simulink model "p1_MCU"  (R2023a)
settings: Solver=FixedStepDiscrete  StartTime=0.0  StopTime=inf  FixedStep=Ts_MCU  RelTol=1e-3  EnableMultiTasking=on
PreLoadFcn:
  | p1_params_new
  | spiDataDefinition
InitFcn:
  | mbd_s32k_consistency_checks(bdroot(gcs));
undefined symbols (not defined in the file or in its folder): ack, cpr_handwheel, cpr_steering, Discrete, DriverInput, DrivetrainLeft, DrivetrainRight, LQFP, MPU_IO, n_handwheel, n_steering, p1data, p1params, param, sr, steering_limit, SteeringLeft, SteeringRight, Time, Ts_MCU, wc, WheelForceLeft, WheelForceRight
libraries: simulink x74, mbd_s32k1xx_ec_toolbox x58, Library_Drivetrain x5, Library_Steering x5, etargetslib x3, ctrlSharedLib x1
(part 1 of 4)
PreSaveFcn:
  | p1_params_new
  | spiDataDefinition
Description:
  | Sample code for extracting X,Y,Z components of acceleration from the on-board sensor.
  | 
  | Extra Modules (In addition to template defaults):
  | LPSPI0 (Accelerometer connection)
  | 
  | For more information, see our Accelerometer Guide:
  | https://www.audesseinc.com/labs/resources/accelerometer-guide/
  | 
  | Revision: 1.2
settings Model: LastModifiedBy=cbeal
settings SolverCC: AlgebraicLoopSolver=TrustRegion
settings DataIOCC: ExternalInput=off  InitialState=off  SaveOutput=off  SignalLogging=off  SaveTime=off
settings OptimizationCC: BlockReduction=off  DefaultParameterBehavior=Inlined  DefaultUnderspecifiedDataType=single  OptimizeBlockIOStorage=off  BufferReuse=off  GlobalBufferReuse=off  ExpressionFolding=off  EnableMemcpy=off  PassReuseOutputArgsAs=Individual arguments  LocalBlockOutputs=off  OptimizeDataStoreBuffers=off  BusAssignmentInplaceUpdate=off  OptimizationLevel=level0  EfficientTunableParamExpr=on
settings DebuggingCC: InheritedTsInSrcMsg=none  SingleTaskRateTransMsg=error  ParameterTunabilityLossMsg=error  UnconnectedInputMsg=error  UnconnectedOutputMsg=error  UnconnectedLineMsg=error  UnknownTsInhSupMsg=error  ArithmeticOperatorsInVariantConditions=warning
settings HardwareCC: ProdBitPerPointer=32  ProdBitPerSizeT=32  ProdBitPerPtrDiffT=32  ProdLargestAtomicInteger=Long  ProdLargestAtomicFloat=Double  ProdWordSize=32  ProdHWDeviceType=ARM Compatible->ARM Cortex
settings ModelReferenceCC: EnableRefExpFcnMdlSchedulingChecks=on
settings SFSimCC: MATLABDynamicMemAlloc=off  CustomCodeUndefinedFunction=UseInterfaceOnly
settings RTWCC: Description=Model Based Design Toolbox S32K1xx Code Generation Target  SystemTargetFile=mbd_s32k.tlc  MakeCommand=mbd_s32k_make_rtw COPY_MDLREF_INCLUDES=0  TemplateMakefile=mbd_s32k.tmf  GenerateReport=on  IncludeHyperlinkInReport=on  LaunchReport=on  GenerateTraceInfo=on  GenerateTraceReport=on  GenerateTraceReportSl=on  GenerateTraceReportSf=on  GenerateTraceReportEml=on  DLArmComputeVersion=19.05
settings CodeAppCC: ForceParamTrailComments=on  IgnoreCustomStorageClasses=off  OperatorAnnotations=on  SimulinkDataObjDesc=on  SFDataObjDesc=on  InsertBlockDesc=on  StateflowObjectComments=on
settings STFCustomTargetCC: MultiwordLength=256  ConcurrentExecutionCompliant=off  CombineOutputUpdateFcns=on  ERTCustomFileBanners=on  SupportContinuousTime=off  RemoveResetFunc=on  MATLABClassNameForMDSCustomization=Simulink.SoftwareTarget.ERTCustomization  GRTInterface=off  UseToolchainInfoCompliant=off  SystemTargetFile=mbd_s32k.tlc
settings ERTTargetCC: TargetLangStandard=C99 (ISO)  ParMdlRefBuildCompliant=off  CompOptLevelCompliant=off  ConcurrentExecutionCompliant=off  SupportNonInlinedSFcns=on  ModelStepFunctionPrototypeControlCompliant=off  CPPClassGenCompliant=off  UseToolchainInfoCompliant=off  InlinedParameterPlacement=NonHierarchical  ERTSrcFileBannerTemplate=mbd_ert_code_template.cgt  ERTHdrFileBannerTemplate=mbd_ert_code_template.cgt  ERTDataSrcFileTemplate=mbd_ert_code_template.cgt  ERTDataHdrFileTemplate=mbd_ert_code_template.cgt  ERTCustomFileTemplate=example_file_process.tlc

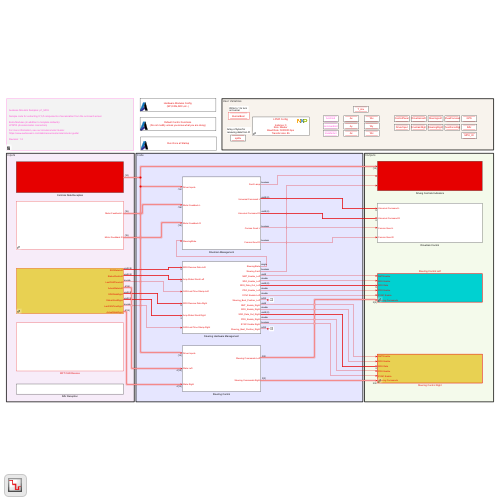
[thumbnail: Simulink's stored preview of the top-level diagram]
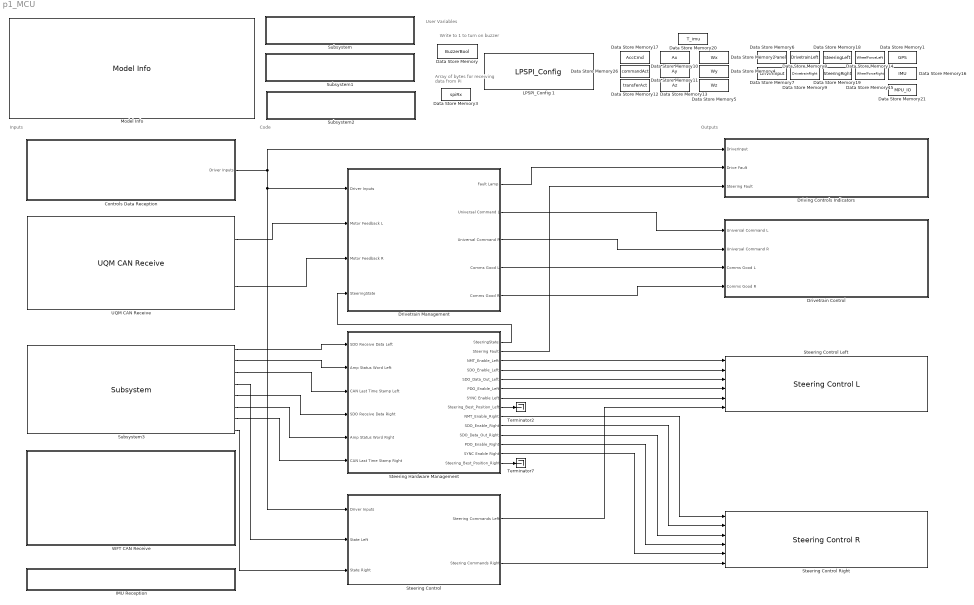
== system p1_MCU ==
  note: User Variables
  note: Write to 1 to turn on buzzer
  note: Inputs
  note: Code
  note: Outputs
  note: Array of bytes for receiving data from Pi
  " Controls Data Reception" : Subsystem  Priority=8
  Data Store Memory : DataStoreMemory  DataStoreName=BuzzerBool  ReadBeforeWriteMsg=warning  WriteAfterWriteMsg=warning  WriteAfterReadMsg=warning  ShowAdditionalParam=off  OutDataTypeStr=boolean
  Data Store Memory1 : DataStoreMemory  DataStoreName=GPS  ReadBeforeWriteMsg=warning  WriteAfterWriteMsg=warning  WriteAfterReadMsg=warning  InitialValue=zeros(p1data.gpsBytes,1)  ShowAdditionalParam=off  OutDataTypeStr=uint8
  Data Store Memory10 : DataStoreMemory  DataStoreName=Ax  ReadBeforeWriteMsg=warning  WriteAfterWriteMsg=warning  WriteAfterReadMsg=warning  InitialValue=[0]  ShowAdditionalParam=off  OutDataTypeStr=single
  Data Store Memory11 : DataStoreMemory  DataStoreName=Ay  ReadBeforeWriteMsg=warning  WriteAfterWriteMsg=warning  WriteAfterReadMsg=warning  InitialValue=[0]  ShowAdditionalParam=off  OutDataTypeStr=single
  Data Store Memory12 : DataStoreMemory  DataStoreName=transferAct  ReadBeforeWriteMsg=warning  WriteAfterWriteMsg=warning  WriteAfterReadMsg=warning  InitialValue=[1]  ShowAdditionalParam=off  OutDataTypeStr=boolean
  Data Store Memory13 : DataStoreMemory  DataStoreName=Az  ReadBeforeWriteMsg=warning  WriteAfterWriteMsg=warning  WriteAfterReadMsg=warning  InitialValue=[0]  ShowAdditionalParam=off  OutDataTypeStr=single
  Data Store Memory14 : DataStoreMemory  DataStoreName=WheelForceLeft  ReadBeforeWriteMsg=warning  WriteAfterWriteMsg=warning  WriteAfterReadMsg=warning  InitialValue=zeros(p1data.wftBytes,1)  ShowAdditionalParam=off  OutDataTypeStr=uint8
  Data Store Memory15 : DataStoreMemory  DataStoreName=WheelForceRight  ReadBeforeWriteMsg=warning  WriteAfterWriteMsg=warning  WriteAfterReadMsg=warning  InitialValue=zeros(p1data.wftBytes,1)  ShowAdditionalParam=off  OutDataTypeStr=uint8
  Data Store Memory16 : DataStoreMemory  DataStoreName=IMU  ReadBeforeWriteMsg=warning  WriteAfterWriteMsg=warning  WriteAfterReadMsg=warning  InitialValue=zeros(p1data.imuBytes,1)  ShowAdditionalParam=off  OutDataTypeStr=uint8
  Data Store Memory17 : DataStoreMemory  DataStoreName=AccCmd  ReadBeforeWriteMsg=warning  WriteAfterWriteMsg=warning  WriteAfterReadMsg=warning  InitialValue=[4436]  ShowAdditionalParam=off  OutDataTypeStr=uint16
  Data Store Memory18 : DataStoreMemory  DataStoreName=SteeringLeft  ReadBeforeWriteMsg=warning  WriteAfterWriteMsg=warning  WriteAfterReadMsg=warning  InitialValue=zeros(p1data.steeringBytes,1)  ShowAdditionalParam=off  OutDataTypeStr=uint8
  Data Store Memory19 : DataStoreMemory  DataStoreName=SteeringRight  ReadBeforeWriteMsg=warning  WriteAfterWriteMsg=warning  WriteAfterReadMsg=warning  InitialValue=zeros(p1data.steeringBytes,1)  ShowAdditionalParam=off  OutDataTypeStr=uint8
  Data Store Memory2 : DataStoreMemory  DataStoreName=Wx  ReadBeforeWriteMsg=warning  WriteAfterWriteMsg=warning  WriteAfterReadMsg=warning  InitialValue=[0]  ShowAdditionalParam=off  OutDataTypeStr=single
  Data Store Memory20 : DataStoreMemory  DataStoreName=T_imu  ReadBeforeWriteMsg=warning  WriteAfterWriteMsg=warning  WriteAfterReadMsg=warning  InitialValue=[0]  ShowAdditionalParam=off  OutDataTypeStr=single
  Data Store Memory21 : DataStoreMemory  DataStoreName=MPU_IO  ReadBeforeWriteMsg=warning  WriteAfterWriteMsg=warning  WriteAfterReadMsg=warning  InitialValue=zeros(p1data.mpuBytes,1)  ShowAdditionalParam=off  OutDataTypeStr=uint8
  Data Store Memory26 : DataStoreMemory  DataStoreName=commandAct  ReadBeforeWriteMsg=warning  WriteAfterWriteMsg=warning  WriteAfterReadMsg=warning  InitialValue=[0]  ShowAdditionalParam=off  OutDataTypeStr=boolean
  Data Store Memory3 : DataStoreMemory  DataStoreName=spiRx  ReadBeforeWriteMsg=warning  WriteAfterWriteMsg=warning  WriteAfterReadMsg=warning  InitialValue=zeros(p1data.spiBytes,1)  ShowAdditionalParam=off  OutDataTypeStr=uint8
  Data Store Memory4 : DataStoreMemory  DataStoreName=Wy  ReadBeforeWriteMsg=warning  WriteAfterWriteMsg=warning  WriteAfterReadMsg=warning  InitialValue=[0]  ShowAdditionalParam=off  OutDataTypeStr=single
  Data Store Memory5 : DataStoreMemory  DataStoreName=Wz  ReadBeforeWriteMsg=warning  WriteAfterWriteMsg=warning  WriteAfterReadMsg=warning  InitialValue=[0]  ShowAdditionalParam=off  OutDataTypeStr=single
  Data Store Memory6 : DataStoreMemory  DataStoreName=ControlPanel  ReadBeforeWriteMsg=warning  WriteAfterWriteMsg=warning  WriteAfterReadMsg=warning  InitialValue=zeros(p1data.controlPanelBytes,1)  ShowAdditionalParam=off  OutDataTypeStr=uint8
  Data Store Memory7 : DataStoreMemory  DataStoreName=DriverInput  ReadBeforeWriteMsg=warning  WriteAfterWriteMsg=warning  WriteAfterReadMsg=warning  InitialValue=zeros(p1data.driverInputBytes,1)  ShowAdditionalParam=off  OutDataTypeStr=uint8
  Data Store Memory8 : DataStoreMemory  DataStoreName=DrivetrainLeft  ReadBeforeWriteMsg=warning  WriteAfterWriteMsg=warning  WriteAfterReadMsg=warning  InitialValue=zeros(p1data.drivetrainBytes,1)  ShowAdditionalParam=off  OutDataTypeStr=uint8
  Data Store Memory9 : DataStoreMemory  DataStoreName=DrivetrainRight  ReadBeforeWriteMsg=warning  WriteAfterWriteMsg=warning  WriteAfterReadMsg=warning  InitialValue=zeros(p1data.drivetrainBytes,1)  ShowAdditionalParam=off  OutDataTypeStr=uint8
  Drivetrain Control : Subsystem
  Drivetrain Management : Subsystem
  Driving Controls Indicators : Subsystem
  IMU Reception : Subsystem
  LPSPI_Config 1 : mbd_s32k1xx_ec_toolbox/Communication Blocks/SPI Blocks/LPSPI_Config   Priority=0  InstanceNumber=0  Role=Master  BaudRate=5000000  ShowAdvanced=on  sin=PTE1: [LPSPI0_SIN | LPSPI Serial Data Input]  sout=PTE2: [LPSPI0_SOUT | LPSPI Serial Data Output]  sck=PTE0: [LPSPI0_SCK | LPSPI Serial Clock I/O]  pcs0=None  pcs1=None  pcs2=PTE6: [LPSPI0_PCS2 | Peripheral Chip Select 2]  pcs3=None  CPHA=1  CPOL=1  BitOrder=MSB first  TransferSize=8  WhichPCS=0  PCSPol=ActiveLow  ContinuousTransfer=off
  Model Info : simulink/Model-Wide Utilities/Model Info  Frame=on  DisplayStringWithTags=|  HorizontalTextAlignment=Left  LeftAlignmentValue=0.02
      | Audesse Simulink Samples: %<ModelName>
      | 
      | %<Description>
  Steering Control : Subsystem
  Steering Control Left : Library_Steering/Steering Control L  SystemSampleTime=-1  VariantActivationTime=update diagram  Latency=0  AutoFrameSizeCalculation=off
  Steering Control Right : Library_Steering/Steering Control R  SystemSampleTime=-1  VariantActivationTime=update diagram  Latency=0  AutoFrameSizeCalculation=off
  Steering Hardware Management : Subsystem
  Subsystem : Subsystem  Priority=1
      mask Display:
      | scl=1/4;
      | patch(scl*[0,52,90,54],scl*[16,55,146,146],[16/255,118/255,188/255],'bottom-left');
      | patch(scl*[0,27,82,77,68],scl*[16,0,42,62,69],[46/255,49/255,146/255],'bottom-left');
      | patch(scl*[89,125,90,68],scl*[16,16,146,91],[0,0,0],'bottom-left');
      | disp('Hardware Modules Config\n(SPI,CAN,ADC,etc..)');
  Subsystem1 : Subsystem
      mask Display:
      | scl=1/4;
      | patch(scl*[0,52,90,54],scl*[16,55,146,146],[16/255,118/255,188/255],'bottom-left');
      | patch(scl*[0,27,82,77,68],scl*[16,0,42,62,69],[46/255,49/255,146/255],'bottom-left');
      | patch(scl*[89,125,90,68],scl*[16,16,146,91],[0,0,0],'bottom-left');
      | disp('Default Control Functions\n(Do not modify unless you know what you are doing)');
  Subsystem2 : Subsystem  Priority=5
      mask Display:
      | scl=1/4;
      | patch(scl*[0,52,90,54],scl*[16,55,146,146],[16/255,118/255,188/255],'bottom-left');
      | patch(scl*[0,27,82,77,68],scl*[16,0,42,62,69],[46/255,49/255,146/255],'bottom-left');
      | patch(scl*[89,125,90,68],scl*[16,16,146,91],[0,0,0],'bottom-left');
      | disp('Run Once at Startup');
  Subsystem3 : Library_Steering/Subsystem  SystemSampleTime=-1  VariantActivationTime=update diagram  Latency=0  AutoFrameSizeCalculation=off
  Terminator2 : Terminator
  Terminator7 : Terminator
  UQM CAN Receive : Library_Drivetrain/UQM CAN Receive  SystemSampleTime=-1  VariantActivationTime=update diagram  Latency=0  AutoFrameSizeCalculation=off
  WFT CAN Receive : Subsystem
  wires:
  Drivetrain Management/5(Comms Good R) -> Drivetrain Control/4(Comms Good R)
  Drivetrain Management/4(Comms Good L) -> Drivetrain Control/3(Comms Good L)
  " Controls Data Reception"/1(Driver Inputs) -> Driving Controls Indicators/1(DriverInput), Steering Control/1(Driver Inputs), Drivetrain Management/1(Driver Inputs)
  Drivetrain Management/2(Universal Command L) -> Drivetrain Control/1(Universal Command L)
  UQM CAN Receive/2 -> Drivetrain Management/3(Motor Feedback R)
  Drivetrain Management/1(Fault Lamp) -> Driving Controls Indicators/2(Drive Fault)
  Drivetrain Management/3(Universal Command R) -> Drivetrain Control/2(Universal Command R)
  UQM CAN Receive/1 -> Drivetrain Management/2(Motor Feedback L)
  Subsystem3/1 -> Steering Hardware Management/1(SDO Receive Data Left)
  Subsystem3/2 -> Steering Hardware Management/2(Amp Status Word Left)
  Subsystem3/3 -> Steering Hardware Management/3(CAN Last Time Stamp Left)
  Subsystem3/4 -> Steering Control/2(State Left)
  Steering Hardware Management/2(Steering Fault) -> Driving Controls Indicators/3(Steering Fault)
  Steering Hardware Management/3(NMT_Enable_Left) -> Steering Control Left/1
  Steering Hardware Management/4(SDO_Enable_Left) -> Steering Control Left/2
  Steering Hardware Management/5(SDO_Data_Out_Left) -> Steering Control Left/3
  Steering Hardware Management/6(PDO_Enable_Left) -> Steering Control Left/4
  Steering Control/1(Steering Commands Left) -> Steering Control Left/6
  Steering Hardware Management/8(Steering_Best_Position_Left) -> Terminator2/1
  Subsystem3/6 -> Steering Hardware Management/5(Amp Status Word Right)
  Subsystem3/8 -> Steering Control/3(State Right)
  Subsystem3/5 -> Steering Hardware Management/4(SDO Receive Data Right)
  Subsystem3/7 -> Steering Hardware Management/6(CAN Last Time Stamp Right)
  Steering Hardware Management/14(Steering_Best_Position_Right) -> Terminator7/1
  Steering Hardware Management/9(NMT_Enable_Right) -> Steering Control Right/1
  Steering Hardware Management/10(SDO_Enable_Right) -> Steering Control Right/2
  Steering Hardware Management/11(SDO_Data_Out_Right) -> Steering Control Right/3
  Steering Hardware Management/12(PDO_Enable_Right) -> Steering Control Right/4
  Steering Hardware Management/1(SteeringState) -> Drivetrain Management/4(SteeringState)
  Steering Control/2(Steering Commands Right) -> Steering Control Right/6
  Steering Hardware Management/7(SYNC Enable Left) -> Steering Control Left/5
  Steering Hardware Management/13(SYNC Enable Right) -> Steering Control Right/5

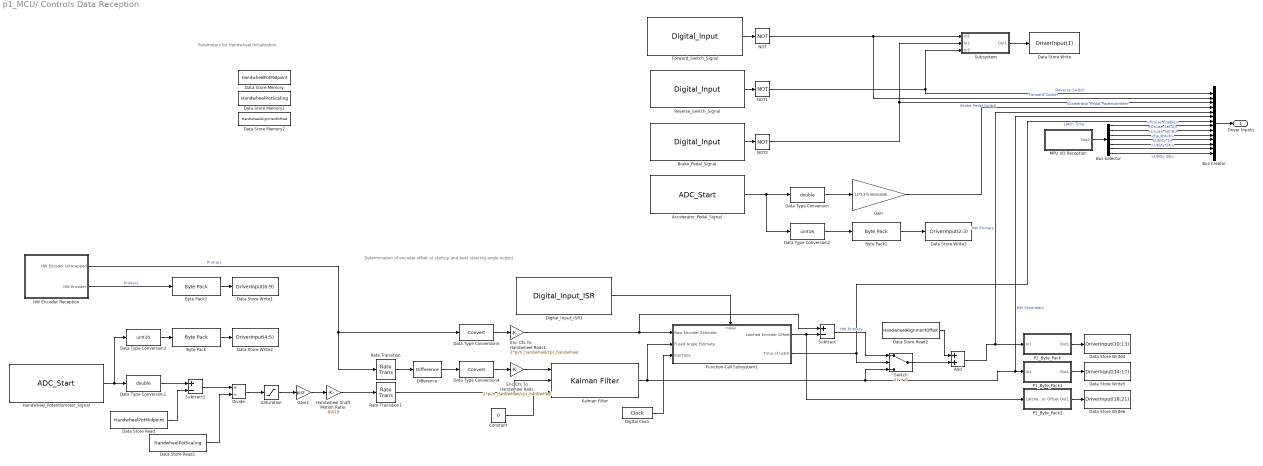
== system p1_MCU/ Controls Data Reception ==
  note: Parameters for Handwheel Initialization
  note: Determination of encoder offset at startup and best steering angle output
  Accelerator_Pedal_Signal : mbd_s32k1xx_ec_toolbox/Motor Control Blocks/ADC Blocks/ADC_Start  instance=1  adc_r=A  adc_chan=PTA15: [ADC1_SE12 | ADC Single Ended Input]  aien=off  mcuTargetUpdate=on
  Add : Sum
  Brake_Pedal_Signal : mbd_s32k1xx_ec_toolbox/GPIO Blocks/Digital_Input  gpio_pin=PTD12: [PTD12 | Port D I/O]  pull_resistor=Pullup  passive_filter=off
  Bus Creator : BusCreator  Inputs=14
  Bus Selector : BusSelector  OutputSignals=Cruise Enable,Cruise Set A,Cruise Set B,Fault Ack,Utility 1,Utility 2A,Utility 2B
  Byte Pack : etargetslib/Byte Pack  datatypes={'uint16'}  byteAlign=1
  Byte Pack1 : etargetslib/Byte Pack  datatypes={'int32'}  byteAlign=1
  Byte Pack2 : etargetslib/Byte Pack  datatypes={'uint16'}  byteAlign=1
  Constant : Constant  Value=0
  Data Store Memory : DataStoreMemory  DataStoreName=HandwheelPotMidpoint  ReadBeforeWriteMsg=warning  WriteAfterWriteMsg=warning  WriteAfterReadMsg=warning  InitialValue=p1params.input.handwheelMidpoint  ShowAdditionalParam=off  OutDataTypeStr=double
  Data Store Memory1 : DataStoreMemory  DataStoreName=HandwheelPotScaling  ReadBeforeWriteMsg=warning  WriteAfterWriteMsg=warning  WriteAfterReadMsg=warning  InitialValue=p1params.input.handwheelScaling  ShowAdditionalParam=off  OutDataTypeStr=double
  Data Store Memory2 : DataStoreMemory  DataStoreName=HandwheelAlignmentOffset  ReadBeforeWriteMsg=warning  WriteAfterWriteMsg=warning  WriteAfterReadMsg=warning  InitialValue=p1params.input.handwheelOffset  ShowAdditionalParam=off  OutDataTypeStr=double
  Data Store Read : DataStoreRead  DataStoreName=HandwheelPotMidpoint  IndexOptions=Index vector (dialog)  Indices=1  OutputSizes=1
  Data Store Read1 : DataStoreRead  DataStoreName=HandwheelPotScaling  IndexOptions=Index vector (dialog)  Indices=1  OutputSizes=1
  Data Store Read2 : DataStoreRead  DataStoreName=HandwheelAlignmentOffset  IndexOptions=Index vector (dialog)  Indices=1  OutputSizes=1
  Data Store Write : DataStoreWrite  DataStoreName=DriverInput  DataStoreElements=DriverInput(1)  IndexOptions=Index vector (dialog)  Indices=1  OutputSizes=1
  Data Store Write1 : DataStoreWrite  DataStoreName=DriverInput  DataStoreElements=DriverInput(6:9)  IndexOptions=Index vector (dialog)  Indices=1  OutputSizes=1
  Data Store Write2 : DataStoreWrite  DataStoreName=DriverInput  DataStoreElements=DriverInput(4:5)  IndexOptions=Index vector (dialog)  Indices=1  OutputSizes=1
  Data Store Write3 : DataStoreWrite  DataStoreName=DriverInput  DataStoreElements=DriverInput(2:3)  IndexOptions=Index vector (dialog)  Indices=1  OutputSizes=1
  Data Store Write4 : DataStoreWrite  DataStoreName=DriverInput  DataStoreElements=DriverInput(10:13)  IndexOptions=Index vector (dialog)  Indices=1  OutputSizes=1
  Data Store Write5 : DataStoreWrite  DataStoreName=DriverInput  DataStoreElements=DriverInput(14:17)  IndexOptions=Index vector (dialog)  Indices=1  OutputSizes=1
  Data Store Write6 : DataStoreWrite  DataStoreName=DriverInput  DataStoreElements=DriverInput(18:21)  IndexOptions=Index vector (dialog)  Indices=1  OutputSizes=1
  Data Type Conversion : DataTypeConversion  OutDataTypeStr=double  SaturateOnIntegerOverflow=off  RndMeth=Floor
  Data Type Conversion1 : DataTypeConversion  OutDataTypeStr=double  SaturateOnIntegerOverflow=off  RndMeth=Floor
  Data Type Conversion2 : DataTypeConversion  OutDataTypeStr=uint16  SaturateOnIntegerOverflow=off  RndMeth=Floor
  Data Type Conversion3 : DataTypeConversion  OutDataTypeStr=uint16  SaturateOnIntegerOverflow=off  RndMeth=Floor
  Data Type Conversion4 : DataTypeConversion  SaturateOnIntegerOverflow=off  RndMeth=Floor
  Data Type Conversion5 : DataTypeConversion  SaturateOnIntegerOverflow=off  RndMeth=Floor
  Difference : simulink/Discrete/Difference  ICPrevInput=0.0  OutMin=[]  OutMax=[]  OutDataType=fixdt(1, 16)  OutScaling=2^-10  DoSatur=off
  Digital Clock : DigitalClock  SampleTime=-1
  Digital_Input_ISR1 : mbd_s32k1xx_ec_toolbox/GPIO Blocks/Digital_Input_ISR  gpio_pin=PTD10: [PTD10 | Port D I/O]  irqc=on either-edge  prio=15
  Divide : Product  Inputs=*/
  Enc Cts To Handwheel Rads : Gain  Gain=2*pi/n_handwheel/cpr_handwheel  SaturateOnIntegerOverflow=on  OutDataTypeStr=Inherit: Same as input  ParamDataTypeStr=Inherit: Same as input
  Enc Cts To Handwheel Rads1 : Gain  Gain=2*pi/n_handwheel/cpr_handwheel  SaturateOnIntegerOverflow=on  OutDataTypeStr=Inherit: Same as input  ParamDataTypeStr=Inherit: Same as input
  Forward_Switch_Signal : mbd_s32k1xx_ec_toolbox/GPIO Blocks/Digital_Input  gpio_pin=PTA0: [PTA0 | Port A I/O]  pull_resistor=Pullup  passive_filter=off
  Function-Call Subsystem1 : Subsystem  TreatAsAtomicUnit=on
  Gain : Gain  Gain=12*3.3*0.9929/4096
  Gain1 : Gain  Gain=pi/2
  HW Encoder Reception : Subsystem
  Handwheel Shaft Motion Ratio : Gain  Gain=-60/18
  Handwheel_Potentiometer_Signal : mbd_s32k1xx_ec_toolbox/Motor Control Blocks/ADC Blocks/ADC_Start  instance=1  adc_r=A  adc_chan=PTB12: [ADC1_SE7 | ADC Single Ended Input]  aien=off  mcuTargetUpdate=on
  Kalman Filter : ctrlSharedLib/Kalman Filter  TimeDomain=Discrete-Time  UseCurrentEstimator=off  ModelSource=Individual A, B, C, D matrices  ModelSourceVariable=ss(0.95,1,1,0,1)  A=1  B=1  C=1  D=0  NumberOfStates=1  NumberOfInputs=1  NumberOfOutputs=1  InitialEstimateSource=Input port  X0=0  P0=10  UseK=off  UseGH=off  NumberOfProcessNoiseInputs=1  G=1  TimeInvariantG=on  H=0  TimeInvariantH=on  Q=0.05  TimeInvariantQ=on  R=50  TimeInvariantR=on  N=0  TimeInvariantN=on  AddInputPort=on  AddEnablePort=off  OutputEstimatedY=off  OutputP=off  Ts=-1
  MPU I/O Reception : Subsystem
  NOT : Logic  Operator=NOT  IconShape=distinctive  AllPortsSameDT=off  OutDataTypeStr=boolean
  NOT1 : Logic  Operator=NOT  IconShape=distinctive  AllPortsSameDT=off  OutDataTypeStr=boolean
  NOT2 : Logic  Operator=NOT  IconShape=distinctive  AllPortsSameDT=off  OutDataTypeStr=boolean
  P1_Byte_Pack : Subsystem
  P1_Byte_Pack1 : Subsystem
  P1_Byte_Pack2 : Subsystem
  Rate Transition : RateTransition  OutPortSampleTime=Ts_MCU
  Rate Transition1 : RateTransition  OutPortSampleTime=Ts_MCU
  Reverse_Switch_Signal : mbd_s32k1xx_ec_toolbox/GPIO Blocks/Digital_Input  gpio_pin=PTD11: [PTD11 | Port D I/O]  pull_resistor=Pullup  passive_filter=off
  Saturation : Saturate  UpperLimit=1  LowerLimit=-1
  Subsystem : Subsystem
  Subtract : Sum  Inputs=+-
  Subtract1 : Sum  Inputs=+-
  Switch : Switch  Criteria=u2 > Threshold  SaturateOnIntegerOverflow=off  InputSameDT=off
  Driver Inputs : Outport
  wires:
  Handwheel_Potentiometer_Signal/1 -> Data Type Conversion3/1, Data Type Conversion1/1
  HW Encoder Reception/2(HW Encoder) -> Byte Pack1/1  "Primary"
  Kalman Filter/1 -> Function-Call Subsystem1/2(Fused Angle Estimate), Switch/3, P1_Byte_Pack1/1(In1), Bus Creator/6  "HW Secondary"
  Gain/1 -> Bus Creator/4  "Accelerator Pedal Potentiometer"
  Brake_Pedal_Signal/1 -> NOT2/1
  Reverse_Switch_Signal/1 -> NOT1/1
  Forward_Switch_Signal/1 -> NOT/1
  NOT/1 -> Bus Creator/2, Subsystem/1(In2)  "Forward Switch"
  Bus Creator/1 -> Driver Inputs/1
  NOT1/1 -> Subsystem/3(In3), Bus Creator/1  "Reverse Switch"
  NOT2/1 -> Subsystem/2(In1), Bus Creator/3  "Brake Pedal Switch"
  Accelerator_Pedal_Signal/1 -> Data Type Conversion2/1, Data Type Conversion/1
  Data Type Conversion/1 -> Gain/1
  Data Type Conversion1/1 -> Subtract1/1
  HW Encoder Reception/1(HW Encoder Unwrapped) -> Data Type Conversion5/1, Rate Transition/1  "Primary"
  Subsystem/1(Out1) -> Data Store Write/1
  Byte Pack/1 -> Data Store Write2/1
  Byte Pack2/1 -> Data Store Write3/1
  Data Type Conversion2/1 -> Byte Pack2/1
  Data Type Conversion3/1 -> Byte Pack/1
  Byte Pack1/1 -> Data Store Write1/1
  Difference/1 -> Data Type Conversion4/1
  Enc Cts To Handwheel Rads/1 -> Kalman Filter/1
  Digital_Input_ISR1/1 -> Function-Call Subsystem1/Trigger
  Switch/1 -> Add/2
  Add/1 -> P1_Byte_Pack/1(In1), Bus Creator/5  "HW Primary"
  Subtract/1 -> Switch/1  "HW Primary"
  Function-Call Subsystem1/2(Time of Latch) -> Switch/2, Bus Creator/7  "Latch Time"
  Rate Transition/1 -> Difference/1
  Rate Transition1/1 -> Kalman Filter/2
  Data Type Conversion4/1 -> Enc Cts To Handwheel Rads/1
  Enc Cts To Handwheel Rads1/1 -> Subtract/1, Function-Call Subsystem1/1(Raw Encoder Estimate)
  Data Type Conversion5/1 -> Enc Cts To Handwheel Rads1/1
  P1_Byte_Pack/1(Out1) -> Data Store Write4/1
  P1_Byte_Pack1/1(Out1) -> Data Store Write5/1
  P1_Byte_Pack2/1(Out1) -> Data Store Write6/1
  Digital Clock/1 -> Function-Call Subsystem1/3(SimTime)
  Function-Call Subsystem1/1(Latched Encoder Offset) -> Subtract/2, P1_Byte_Pack2/1(Latched Encoder Offset)
  Data Store Read1/1 -> Divide/2
  Subtract1/1 -> Divide/1
  Divide/1 -> Saturation/1
  Handwheel Shaft Motion Ratio/1 -> Rate Transition1/1
  Saturation/1 -> Gain1/1
  Data Store Read/1 -> Subtract1/2
  Gain1/1 -> Handwheel Shaft Motion Ratio/1
  Constant/1 -> Kalman Filter/3
  Data Store Read2/1 -> Add/1
  MPU I/O Reception/1(Out1) -> Bus Selector/1
  Bus Selector/1 -> Bus Creator/8  "<Cruise Enable>"
  Bus Selector/2 -> Bus Creator/9  "<Cruise Set A>"
  Bus Selector/3 -> Bus Creator/10  "<Cruise Set B>"
  Bus Selector/4 -> Bus Creator/11  "<Fault Ack>"
  Bus Selector/5 -> Bus Creator/12  "<Utility 1>"
  Bus Selector/6 -> Bus Creator/13  "<Utility 2A>"
  Bus Selector/7 -> Bus Creator/14  "<Utility 2B>"

== system p1_MCU/Drivetrain Control ==
  note: UQM Universal Command - Torque Mode
  note: High Voltage Control Signal
      | (enabled when CAN communication with UQM inverters good)
  note: High Voltage Control Signal
      | (enabled when CAN communication with UQM inverters good)
  Universal Command L : Inport
  Universal Command R : Inport  Port=2
  Comms Good L : Inport  Port=3
  Comms Good R : Inport  Port=4
  CAN_Comms_Established_Signal_(L) : mbd_s32k1xx_ec_toolbox/GPIO Blocks/Digital_Output  Commented=on  gpio_pin=PTD8: [PTD8 | Port D I/O]  init_val=High  drive_strength=Low
  CAN_Comms_Established_Signal_(L)1 : mbd_s32k1xx_ec_toolbox/GPIO Blocks/Digital_Output  gpio_pin=PTD9: [PTD9 | Port D I/O]  init_val=Low  drive_strength=Low
  CAN_Comms_Established_Signal_(R) : mbd_s32k1xx_ec_toolbox/GPIO Blocks/Digital_Output  Commented=on  gpio_pin=PTE15: [PTE15 | Port E I/O]  init_val=High  drive_strength=Low
  CAN_Comms_Established_Signal_(R)1 : mbd_s32k1xx_ec_toolbox/GPIO Blocks/Digital_Output  gpio_pin=PTE16: [PTE16 | Port E I/O]  init_val=High  drive_strength=Low
  FCAN_Transfer_Status1 : mbd_s32k1xx_ec_toolbox/Communication Blocks/CAN Blocks/FCAN_Transfer_Status  can_instance=1  can_mb_idx=4
  FCAN_Transfer_Status3 : mbd_s32k1xx_ec_toolbox/Communication Blocks/CAN Blocks/FCAN_Transfer_Status  can_instance=1  can_mb_idx=3
  If Action Subsystem1 : Library_Drivetrain/If Action Subsystem1  SystemSampleTime=-1  VariantActivationTime=update diagram  Latency=0  AutoFrameSizeCalculation=off
  If Action Subsystem3 : Library_Drivetrain/If Action Subsystem3  SystemSampleTime=-1  VariantActivationTime=update diagram  Latency=0  AutoFrameSizeCalculation=off
  If1 : If  IfExpression=u1 == 0  ShowElse=off
  If3 : If  IfExpression=u1 == 0  ShowElse=off
  NOT1 : Logic  Commented=on  Operator=NOT  IconShape=distinctive  AllPortsSameDT=off  OutDataTypeStr=boolean
  NOT2 : Logic  Commented=on  Operator=NOT  IconShape=distinctive  AllPortsSameDT=off  OutDataTypeStr=boolean
  wires:
  FCAN_Transfer_Status1/1 -> If1/1
  Universal Command L/1 -> If Action Subsystem3/1
  If1/1 -> If Action Subsystem1/Action
  If3/1 -> If Action Subsystem3/Action
  Universal Command R/1 -> If Action Subsystem1/1
  FCAN_Transfer_Status3/1 -> If3/1
  NOT1/1 -> CAN_Comms_Established_Signal_(R)/1
  NOT2/1 -> CAN_Comms_Established_Signal_(L)/1
  Comms Good L/1 -> CAN_Comms_Established_Signal_(L)1/1
  Comms Good R/1 -> CAN_Comms_Established_Signal_(R)1/1

== system p1_MCU/Drivetrain Management ==
  Driver Inputs : Inport
  Motor Feedback L : Inport  Port=2
  Motor Feedback R : Inport  Port=3
  SteeringState : Inport  Port=4
  1-D Lookup Table : Lookup_n-D  NumberOfTableDimensions=1  BreakpointsForDimension1="[0 p1params.input.VminAccel p1params.input.VmidAccel-p1params.input.Vdeadband/2  p1params.input.VmidAccel+p1params.input.Vdeadband/2 p1params.input.VmaxAccel 5]"  Table=[p1params.input.TmaxAccel p1params.input.TmaxAccel 0 0 p1params.input.TminAccel p1params.input.TminAccel]  InternalRulePriority=Speed  RndMeth=Simplest
  Bus Selector : BusSelector  OutputSignals=Accelerator Pedal Potentiometer
  Bus Selector2 : BusSelector  OutputSignals=UQM Feedback L.Speed Left,Status Bytes L,Last CAN Time L
  Bus Selector3 : BusSelector  OutputSignals=Reverse Switch
  Bus Selector4 : BusSelector  OutputSignals=UQM Feedback R.Speed Right,Status Bytes R,Last CAN Time R
  Data Store Memory1 : DataStoreMemory  DataStoreName=param_VelLimFWD  ReadBeforeWriteMsg=warning  WriteAfterWriteMsg=warning  WriteAfterReadMsg=warning  InitialValue=p1params.drivetrain.left.velLimFWD  ShowAdditionalParam=off  OutDataTypeStr=double
  Data Store Memory2 : DataStoreMemory  DataStoreName=param_VelLimREV  ReadBeforeWriteMsg=warning  WriteAfterWriteMsg=warning  WriteAfterReadMsg=warning  InitialValue=p1params.drivetrain.left.velLimREV  ShowAdditionalParam=off  OutDataTypeStr=double
  Data Store Read : DataStoreRead  DataStoreName=param_VelLimFWD  IndexOptions=Index vector (dialog)  Indices=1  OutputSizes=1
  Data Store Read1 : DataStoreRead  DataStoreName=param_VelLimREV  IndexOptions=Index vector (dialog)  Indices=1  OutputSizes=1
  Delay : Delay  DelayLength=1
  Delay1 : Delay  DelayLength=1
  Discrete FIR Filter : DiscreteFir  Coefficients=[ones(1,20)/20]
  Gain : Gain
  OR : Logic  Operator=OR  IconShape=distinctive  AllPortsSameDT=off  OutDataTypeStr=boolean
  Subsystem : Subsystem
  Subsystem1 : Subsystem
  Switch : Switch  Criteria=u2 > Threshold  SaturateOnIntegerOverflow=off  InputSameDT=off
  Wheel Circumference1 : Gain  Gain=2*pi*0.3/5.6
  Wheel Circumference3 : Gain  Gain=2*pi*0.3/5.6
  Fault Lamp : Outport
  Universal Command L : Outport  Port=2
  Universal Command R : Outport  Port=3
  Comms Good L : Outport  Port=4
  Comms Good R : Outport  Port=5
  wires:
  Data Store Read/1 -> Subsystem/3(Pos Velocity Lim), Subsystem1/3(Pos Velocity Lim)
  Subsystem/3(Comms Good Flag) -> Delay/1, Comms Good L/1  "MotorCommsGoodLeft"
  Data Store Read1/1 -> Subsystem/4(Neg Velocity Lim), Subsystem1/4(Neg Velocity Lim)
  SteeringState/1 -> Subsystem1/5(Steering Mode), Subsystem/5(Steering Mode)
  Bus Selector4/1 -> Wheel Circumference1/1  "<Speed Right>"
  1-D Lookup Table/1 -> Switch/3, Gain/1  "TorqueRequest"
  Bus Selector/1 -> Discrete FIR Filter/1  "<Accelerator Pedal Potentiometer>"
  Wheel Circumference1/1 -> Subsystem1/7(Vehicle Speed)
  Subsystem1/1(Drive Fault Lamp) -> OR/2
  Subsystem/2(Universal Command) -> Universal Command L/1  "UnivCmdLeft"
  Subsystem1/2(Universal Command) -> Universal Command R/1  "UnivCmdRight"
  Driver Inputs/1 -> Subsystem/1(Driver Controls), Bus Selector3/1, Subsystem1/1(Driver Controls), Bus Selector/1
  Motor Feedback R/1 -> Bus Selector4/1
  Subsystem1/3(Comms Good Flag) -> Comms Good R/1, Delay1/1
  OR/1 -> Fault Lamp/1
  Subsystem/1(Drive Fault Lamp) -> OR/1
  Delay/1 -> Subsystem1/6(Comms Good (Opposing Motor))
  Delay1/1 -> Subsystem/6(Comms Good (Opposing Motor))
  Switch/1 -> Subsystem1/2(Torque Request), Subsystem/2(Torque Request)
  Bus Selector3/1 -> Switch/2  "<Reverse Switch>"
  Gain/1 -> Switch/1
  Bus Selector4/2 -> Subsystem1/8(Motor Feedback)  "<Status Bytes R>"
  Bus Selector4/3 -> Subsystem1/9(Last CAN Time)  "<Last CAN Time R>"
  Bus Selector2/2 -> Subsystem/8(Motor Feedback)  "<Status Bytes L>"
  Bus Selector2/3 -> Subsystem/9(Last CAN Time)  "<Last CAN Time L>"
  Motor Feedback L/1 -> Bus Selector2/1
  Bus Selector2/1 -> Wheel Circumference3/1  "<Speed Left>"
  Wheel Circumference3/1 -> Subsystem/7(Vehicle Speed)
  Discrete FIR Filter/1 -> 1-D Lookup Table/1

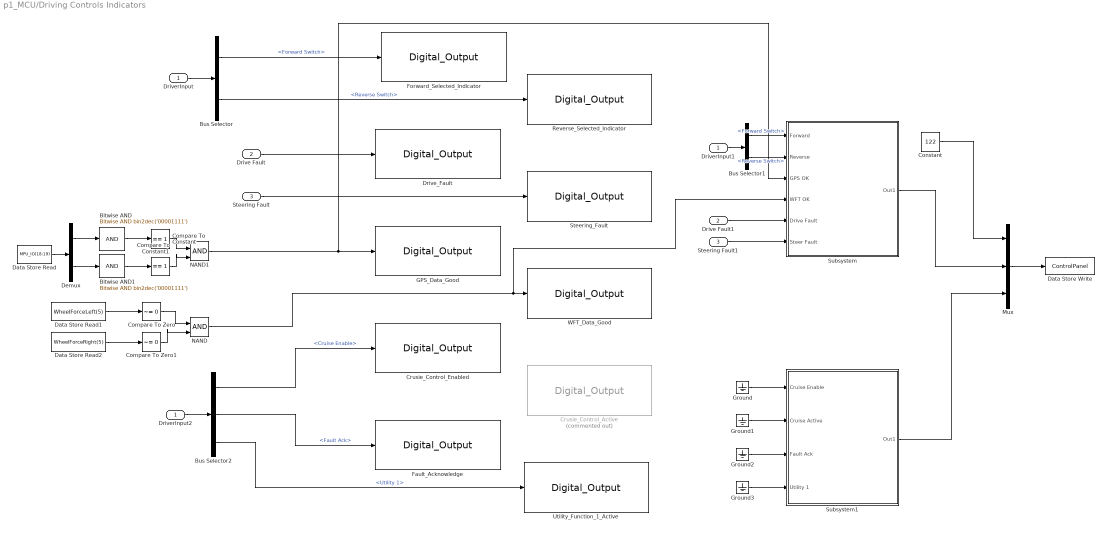
== system p1_MCU/Driving Controls Indicators ==
  DriverInput : Inport
  Drive Fault : Inport  Port=2
  Steering Fault : Inport  Port=3
  Bitwise AND : simulink/Logic and Bit Operations/Bitwise Operator  logicop=AND  UseBitMask=on  BitMask=bin2dec('00001111')  BitMaskRealWorld=Stored Integer
  Bitwise AND1 : simulink/Logic and Bit Operations/Bitwise Operator  logicop=AND  UseBitMask=on  BitMask=bin2dec('00001111')  BitMaskRealWorld=Stored Integer
  Bus Selector : BusSelector  OutputSignals=Forward Switch,Reverse Switch
  Bus Selector1 : BusSelector  OutputSignals=Forward Switch,Reverse Switch
  Bus Selector2 : BusSelector  OutputSignals=Cruise Enable,Fault Ack,Utility 1
  Compare To Constant : simulink/Logic and Bit Operations/Compare To Constant  relop===  const=1  OutDataTypeStr=boolean
  Compare To Constant1 : simulink/Logic and Bit Operations/Compare To Constant  relop===  const=1  OutDataTypeStr=boolean
  Compare To Zero : simulink/Logic and Bit Operations/Compare To Zero  relop=~=  OutDataTypeStr=boolean
  Compare To Zero1 : simulink/Logic and Bit Operations/Compare To Zero  relop=~=  OutDataTypeStr=boolean
  Constant : Constant  Value=122  OutDataTypeStr=uint8
  Crusie_Control_Active : mbd_s32k1xx_ec_toolbox/GPIO Blocks/Digital_Output  Commented=on  gpio_pin=PTE5: [PTE5 | Port E I/O]  init_val=Low  drive_strength=Low
  Crusie_Control_Enabled : mbd_s32k1xx_ec_toolbox/GPIO Blocks/Digital_Output  gpio_pin=PTB11: [PTB11 | Port B I/O]  init_val=Low  drive_strength=Low
  Data Store Read : DataStoreRead  DataStoreName=MPU_IO  DataStoreElements=MPU_IO(18:19)  IndexOptions=Index vector (dialog)  Indices=1  OutputSizes=1
  Data Store Read1 : DataStoreRead  DataStoreName=WheelForceLeft  DataStoreElements=WheelForceLeft(5)  IndexOptions=Index vector (dialog)  Indices=1  OutputSizes=1
  Data Store Read2 : DataStoreRead  DataStoreName=WheelForceRight  DataStoreElements=WheelForceRight(5)  IndexOptions=Index vector (dialog)  Indices=1  OutputSizes=1
  Data Store Write : DataStoreWrite  DataStoreName=ControlPanel  IndexOptions=Index vector (dialog)  Indices=1  OutputSizes=1
  Demux : Demux  Outputs=2
  Drive Fault1 : InportShadow  Port=2
  Drive_Fault : mbd_s32k1xx_ec_toolbox/GPIO Blocks/Digital_Output  gpio_pin=PTD3: [PTD3 | Port D I/O]  init_val=Low  drive_strength=Low
  DriverInput1 : InportShadow
  DriverInput2 : InportShadow
  Fault_Acknowledge : mbd_s32k1xx_ec_toolbox/GPIO Blocks/Digital_Output  gpio_pin=PTE5: [PTE5 | Port E I/O]  init_val=Low  drive_strength=Low
  Forward_Selected_Indicator : mbd_s32k1xx_ec_toolbox/GPIO Blocks/Digital_Output  gpio_pin=PTD1: [PTD1 | Port D I/O]  init_val=Low  drive_strength=Low
  GPS_Data_Good : mbd_s32k1xx_ec_toolbox/GPIO Blocks/Digital_Output  gpio_pin=PTE9: [PTE9 | Port E I/O]  init_val=Low  drive_strength=Low
  Ground{,1..3} (4 alike) : Ground
  Mux : Mux  Inputs=3
  NAND : Logic  IconShape=distinctive  AllPortsSameDT=off  OutDataTypeStr=boolean
  NAND1 : Logic  IconShape=distinctive  AllPortsSameDT=off  OutDataTypeStr=boolean
  Reverse_Selected_Indicator : mbd_s32k1xx_ec_toolbox/GPIO Blocks/Digital_Output  gpio_pin=PTC13: [PTC13 | Port C I/O]  init_val=Low  drive_strength=Low
  Steering Fault1 : InportShadow  Port=3
  Steering_Fault : mbd_s32k1xx_ec_toolbox/GPIO Blocks/Digital_Output  gpio_pin=PTE11: [PTE11 | Port E I/O]  init_val=Low  drive_strength=Low
  Subsystem : Subsystem
  Subsystem1 : Subsystem
  Utility_Function_1_Active : mbd_s32k1xx_ec_toolbox/GPIO Blocks/Digital_Output  gpio_pin=PTB5: [PTB5 | Port B I/O]  init_val=Low  drive_strength=Low
  WFT_Data_Good : mbd_s32k1xx_ec_toolbox/GPIO Blocks/Digital_Output  gpio_pin=PTC15: [PTC15 | Port C I/O]  init_val=Low  drive_strength=Low
  wires:
  DriverInput/1 -> Bus Selector/1
  Bus Selector/2 -> Reverse_Selected_Indicator/1  "<Reverse Switch>"
  Drive Fault/1 -> Drive_Fault/1
  Steering Fault/1 -> Steering_Fault/1
  Subsystem/1(Out1) -> Mux/2
  DriverInput1/1 -> Bus Selector1/1
  Bus Selector1/1 -> Subsystem/1(Forward)  "<Forward Switch>"
  Bus Selector1/2 -> Subsystem/2(Reverse)  "<Reverse Switch>"
  Drive Fault1/1 -> Subsystem/5(Drive Fault)
  Steering Fault1/1 -> Subsystem/6(Steer Fault)
  NAND1/1 -> Subsystem/3(GPS OK), GPS_Data_Good/1
  Subsystem1/1(Out1) -> Mux/3
  Ground/1 -> Subsystem1/1(Cruise Enable)
  Ground1/1 -> Subsystem1/2(Cruise Active)
  Ground2/1 -> Subsystem1/3(Fault Ack)
  Ground3/1 -> Subsystem1/4(Utility 1)
  NAND/1 -> WFT_Data_Good/1, Subsystem/4(WFT OK)
  Data Store Read2/1 -> Compare To Zero1/1
  Data Store Read1/1 -> Compare To Zero/1
  Compare To Zero/1 -> NAND/1
  Compare To Zero1/1 -> NAND/2
  Bus Selector/1 -> Forward_Selected_Indicator/1  "<Forward Switch>"
  DriverInput2/1 -> Bus Selector2/1
  Bus Selector2/1 -> Crusie_Control_Enabled/1  "<Cruise Enable>"
  Bus Selector2/2 -> Fault_Acknowledge/1  "<Fault Ack>"
  Bus Selector2/3 -> Utility_Function_1_Active/1  "<Utility 1>"
  Data Store Read/1 -> Demux/1
  Demux/1 -> Bitwise AND/1
  Bitwise AND/1 -> Compare To Constant/1
  Demux/2 -> Bitwise AND1/1
  Bitwise AND1/1 -> Compare To Constant1/1
  Compare To Constant/1 -> NAND1/1
  Compare To Constant1/1 -> NAND1/2
  Mux/1 -> Data Store Write/1
  Constant/1 -> Mux/1

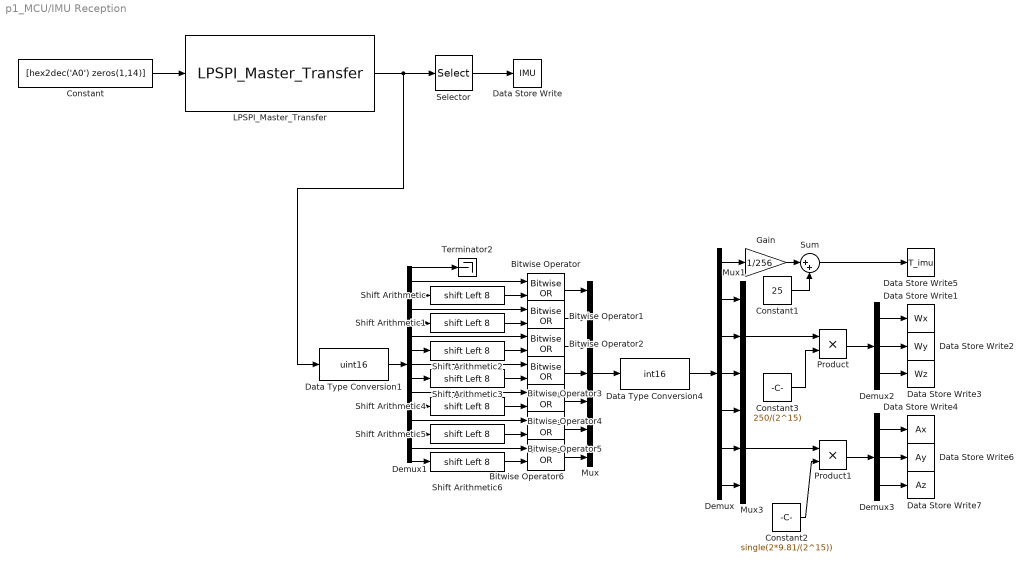
== system p1_MCU/IMU Reception ==
  Bitwise Operator{,1..6} (7 alike) : simulink/Logic and Bit Operations/Bitwise Operator  logicop=OR  UseBitMask=off  NumInputPorts=2  BitMask=bin2dec('11011001')  BitMaskRealWorld=Stored Integer
  Constant : Constant  Value=[hex2dec('A0') zeros(1,14)]  OutDataTypeStr=uint8
  Constant1 : Constant  Value=25  OutDataTypeStr=single
  Constant2 : Constant  Value=single(2*9.81/(2^15))  OutDataTypeStr=single
  Constant3 : Constant  Value=250/(2^15)  OutDataTypeStr=Inherit: Inherit via back propagation
  Data Store Write : DataStoreWrite  DataStoreName=IMU  IndexOptions=Index vector (dialog)  Indices=1  OutputSizes=1
  Data Store Write1 : DataStoreWrite  DataStoreName=Wx  IndexOptions=Index vector (dialog)  Indices=1  OutputSizes=1
  Data Store Write2 : DataStoreWrite  DataStoreName=Wy  IndexOptions=Index vector (dialog)  Indices=1  OutputSizes=1
  Data Store Write3 : DataStoreWrite  DataStoreName=Wz  IndexOptions=Index vector (dialog)  Indices=1  OutputSizes=1
  Data Store Write4 : DataStoreWrite  DataStoreName=Ax  IndexOptions=Index vector (dialog)  Indices=1  OutputSizes=1
  Data Store Write5 : DataStoreWrite  DataStoreName=T_imu  IndexOptions=Index vector (dialog)  Indices=1  OutputSizes=1
  Data Store Write6 : DataStoreWrite  DataStoreName=Ay  IndexOptions=Index vector (dialog)  Indices=1  OutputSizes=1
  Data Store Write7 : DataStoreWrite  DataStoreName=Az  IndexOptions=Index vector (dialog)  Indices=1  OutputSizes=1
  Data Type Conversion1 : DataTypeConversion  OutDataTypeStr=uint16  SaturateOnIntegerOverflow=off  RndMeth=Floor
  Data Type Conversion4 : DataTypeConversion  OutDataTypeStr=int16  SaturateOnIntegerOverflow=off  RndMeth=Floor
  Demux : Demux  Outputs=7
  Demux1 : Demux  Outputs=15
  Demux2 : Demux  Outputs=3
  Demux3 : Demux  Outputs=3
  Gain : Gain  Gain=1/256  OutDataTypeStr=single
  LPSPI_Master_Transfer : mbd_s32k1xx_ec_toolbox/Communication Blocks/SPI Blocks/LPSPI_Master_Transfer  instance=0  pcs=2  pcs_polarity=ActiveLow  xfermode=Non blocking  timeout=50  spi_upd=on
  Mux : Mux  Inputs=7
  Mux1 : Mux  Inputs=3
  Mux3 : Mux  Inputs=3
  Product : Product
  Product1 : Product
  Selector : Selector  InputPortWidth=15  IndexOptions=Index vector (dialog)  Indices=[4:15]  OutputSizes=12
  Shift Arithmetic{,1..6} (7 alike) : ArithShift  BitShiftNumber=8  BitShiftDirection=Left
  Sum : Sum  Inputs=|++
  Terminator2 : Terminator
  wires:
  Selector/1 -> Data Store Write/1
  Constant/1 -> LPSPI_Master_Transfer/1
  LPSPI_Master_Transfer/1 -> Data Type Conversion1/1, Selector/1
  Demux/7 -> Mux3/3
  Constant3/1 -> Product/2
  Demux1/15 -> Shift Arithmetic6/1
  Demux2/3 -> Data Store Write3/1
  Mux1/1 -> Product/1
  Shift Arithmetic4/1 -> Bitwise Operator4/2
  Demux1/13 -> Shift Arithmetic5/1
  Product1/1 -> Demux3/1
  Shift Arithmetic5/1 -> Bitwise Operator5/2
  Shift Arithmetic2/1 -> Bitwise Operator2/2
  Demux3/2 -> Data Store Write6/1
  Bitwise Operator/1 -> Mux/1
  Demux3/1 -> Data Store Write4/1
  Constant1/1 -> Sum/2
  Demux1/11 -> Shift Arithmetic4/1
  Gain/1 -> Sum/1
  Demux1/7 -> Shift Arithmetic2/1
  Bitwise Operator3/1 -> Mux/4
  Mux3/1 -> Product1/1
  Product/1 -> Demux2/1
  Constant2/1 -> Product1/2
  Demux/5 -> Mux3/1
  Demux1/4 -> Bitwise Operator1/1
  Bitwise Operator2/1 -> Mux/3
  Demux2/1 -> Data Store Write1/1
  Bitwise Operator5/1 -> Mux/6
  Demux/3 -> Mux1/2
  Demux/6 -> Mux3/2
  Demux/1 -> Gain/1
  Bitwise Operator4/1 -> Mux/5
  Demux/4 -> Mux1/3
  Demux1/2 -> Bitwise Operator/1
  Shift Arithmetic6/1 -> Bitwise Operator6/2
  Demux1/5 -> Shift Arithmetic1/1
  Demux1/14 -> Bitwise Operator6/1
  Bitwise Operator6/1 -> Mux/7
  Demux1/1 -> Terminator2/1
  Bitwise Operator1/1 -> Mux/2
  Demux1/12 -> Bitwise Operator5/1
  Shift Arithmetic1/1 -> Bitwise Operator1/2
  Demux2/2 -> Data Store Write2/1
  Data Type Conversion1/1 -> Demux1/1
  Sum/1 -> Data Store Write5/1
  Data Type Conversion4/1 -> Demux/1
  Shift Arithmetic3/1 -> Bitwise Operator3/2
  Demux1/8 -> Bitwise Operator3/1
  Mux/1 -> Data Type Conversion4/1
  Demux1/6 -> Bitwise Operator2/1
  Demux1/10 -> Bitwise Operator4/1
  Demux1/3 -> Shift Arithmetic/1
  Demux3/3 -> Data Store Write7/1
  Shift Arithmetic/1 -> Bitwise Operator/2
  Demux1/9 -> Shift Arithmetic3/1
  Demux/2 -> Mux1/1

== system p1_MCU/Steering Control ==
  Driver Inputs : Inport
  State Left : Inport  Port=2
  State Right : Inport  Port=3
  Bias : Bias  SaturateOnIntegerOverflow=off
  Bias1 : Bias  SaturateOnIntegerOverflow=off
  Bus Creator : BusCreator  Inputs=3
  Bus Creator1 : BusCreator  Inputs=3
  Constant{,1..4} (5 alike) : Constant  Value=0
  Demux : Demux  Outputs=2
  Gain : Gain  Gain=n_steering*cpr_steering/(2*pi)
  Position Soft Limits (Left) : Saturate  UpperLimit=55000  LowerLimit=-45000  OutDataTypeStr=Inherit: Inherit via back propagation
  Position Soft Limits (Right) : Saturate  UpperLimit=55000  LowerLimit=-55000  OutDataTypeStr=Inherit: Inherit via back propagation
  Steering Controller : Subsystem
      mask init:
      | p1_params_new;
      | SteeringController;
  Terminator : Terminator
  Terminator1 : Terminator
  Steering Commands Left : Outport
  Steering Commands Right : Outport  Port=2
  wires:
  Position Soft Limits (Left)/1 -> Bias/1  "Target Angle"
  Driver Inputs/1 -> Steering Controller/1(Driver Input)
  Bus Creator/1 -> Steering Commands Left/1
  Bus Creator1/1 -> Steering Commands Right/1
  Position Soft Limits (Right)/1 -> Bias1/1  "Target Angle"
  Constant/1 -> Steering Controller/2(Steering Addition)
  Steering Controller/1(Steering Angle Commands) -> Gain/1
  Demux/1 -> Position Soft Limits (Left)/1
  Demux/2 -> Position Soft Limits (Right)/1
  Constant1/1 -> Bus Creator/2  "Velocity Feedforward"
  Constant2/1 -> Bus Creator/3  "Current Feedforward"
  Constant4/1 -> Bus Creator1/3  "Current Feedforward"
  Constant3/1 -> Bus Creator1/2  "Velocity Feedforward"
  State Left/1 -> Terminator/1
  State Right/1 -> Terminator1/1
  Gain/1 -> Demux/1
  Bias/1 -> Bus Creator/1  "Target Angle"
  Bias1/1 -> Bus Creator1/1  "Target Angle"

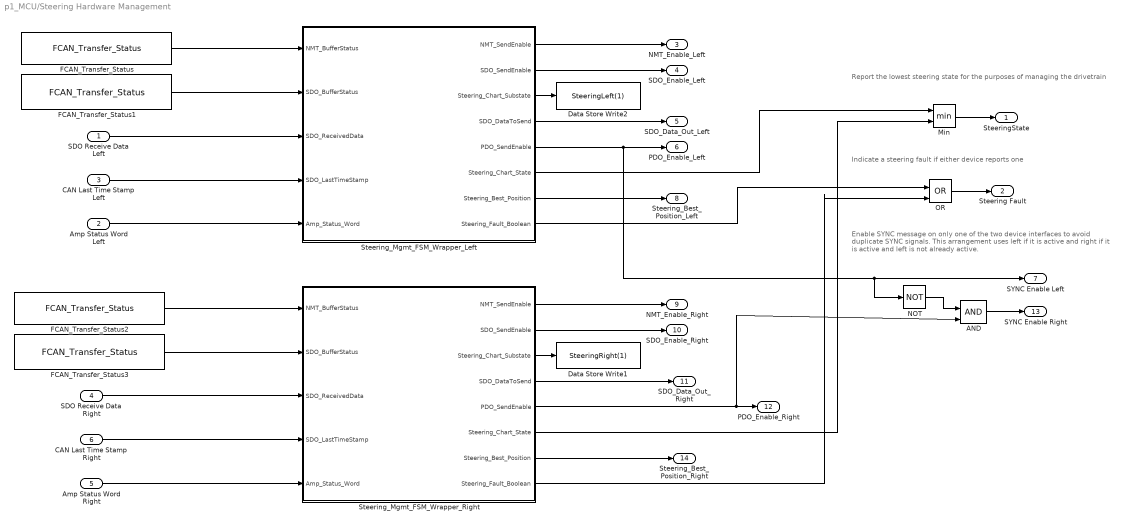
== system p1_MCU/Steering Hardware Management ==
  note: Report the lowest steering state for the purposes of
      | managing the drivetrain
  note: Indicate a steering fault if either device reports one
  note: Enable SYNC message on only one of the two device
      | interfaces to avoid duplicate SYNC signals. This
      | arrangement uses left if it is active and right if it is active
      | and left is not already active.
  SDO Receive Data Left : Inport
  Amp Status Word Left : Inport  Port=2
  CAN Last Time Stamp Left : Inport  Port=3
  SDO Receive Data Right : Inport  Port=4
  Amp Status Word Right : Inport  Port=5
  CAN Last Time Stamp Right : Inport  Port=6
  AND : Logic  IconShape=distinctive  AllPortsSameDT=off  OutDataTypeStr=boolean
  Data Store Write1 : DataStoreWrite  DataStoreName=SteeringRight  DataStoreElements=SteeringRight(1)  IndexOptions=Index vector (dialog)  Indices=1  OutputSizes=1
  Data Store Write2 : DataStoreWrite  DataStoreName=SteeringLeft  DataStoreElements=SteeringLeft(1)  IndexOptions=Index vector (dialog)  Indices=1  OutputSizes=1
  FCAN_Transfer_Status : mbd_s32k1xx_ec_toolbox/Communication Blocks/CAN Blocks/FCAN_Transfer_Status  can_instance=0  can_mb_idx=1
  FCAN_Transfer_Status1 : mbd_s32k1xx_ec_toolbox/Communication Blocks/CAN Blocks/FCAN_Transfer_Status  can_instance=0  can_mb_idx=3
  FCAN_Transfer_Status2 : mbd_s32k1xx_ec_toolbox/Communication Blocks/CAN Blocks/FCAN_Transfer_Status  can_instance=0  can_mb_idx=7
  FCAN_Transfer_Status3 : mbd_s32k1xx_ec_toolbox/Communication Blocks/CAN Blocks/FCAN_Transfer_Status  can_instance=0  can_mb_idx=9
  Min : MinMax  Inputs=2  OutDataTypeStr=single
  NOT : Logic  Operator=NOT  IconShape=distinctive  AllPortsSameDT=off  OutDataTypeStr=boolean
  OR : Logic  Operator=OR  IconShape=distinctive  AllPortsSameDT=off  OutDataTypeStr=boolean
  Steering_Mgmt_FSM_Wrapper_Left : Subsystem
  Steering_Mgmt_FSM_Wrapper_Right : Subsystem
  SteeringState : Outport
  Steering Fault : Outport  Port=2
  NMT_Enable_Left : Outport  Port=3
  SDO_Enable_Left : Outport  Port=4
  SDO_Data_Out_Left : Outport  Port=5
  PDO_Enable_Left : Outport  Port=6
  SYNC Enable Left : Outport  Port=7
  Steering_Best_Position_Left : Outport  Port=8
  NMT_Enable_Right : Outport  Port=9
  SDO_Enable_Right : Outport  Port=10
  SDO_Data_Out_Right : Outport  Port=11
  PDO_Enable_Right : Outport  Port=12
  SYNC Enable Right : Outport  Port=13
  Steering_Best_Position_Right : Outport  Port=14
  wires:
  FCAN_Transfer_Status/1 -> Steering_Mgmt_FSM_Wrapper_Left/1(NMT_BufferStatus)
  FCAN_Transfer_Status1/1 -> Steering_Mgmt_FSM_Wrapper_Left/2(SDO_BufferStatus)
  SDO Receive Data Left/1 -> Steering_Mgmt_FSM_Wrapper_Left/3(SDO_ReceivedData)
  CAN Last Time Stamp Left/1 -> Steering_Mgmt_FSM_Wrapper_Left/4(SDO_LastTimeStamp)
  Steering_Mgmt_FSM_Wrapper_Left/1(NMT_SendEnable) -> NMT_Enable_Left/1
  Steering_Mgmt_FSM_Wrapper_Left/2(SDO_SendEnable) -> SDO_Enable_Left/1
  Steering_Mgmt_FSM_Wrapper_Left/3(Steering_Chart_Substate) -> Data Store Write2/1
  Steering_Mgmt_FSM_Wrapper_Left/4(SDO_DataToSend) -> SDO_Data_Out_Left/1
  Steering_Mgmt_FSM_Wrapper_Left/6(Steering_Chart_State) -> Min/1
  OR/1 -> Steering Fault/1
  Steering_Mgmt_FSM_Wrapper_Left/7(Steering_Best_Position) -> Steering_Best_Position_Left/1
  FCAN_Transfer_Status2/1 -> Steering_Mgmt_FSM_Wrapper_Right/1(NMT_BufferStatus)
  FCAN_Transfer_Status3/1 -> Steering_Mgmt_FSM_Wrapper_Right/2(SDO_BufferStatus)
  SDO Receive Data Right/1 -> Steering_Mgmt_FSM_Wrapper_Right/3(SDO_ReceivedData)
  CAN Last Time Stamp Right/1 -> Steering_Mgmt_FSM_Wrapper_Right/4(SDO_LastTimeStamp)
  Steering_Mgmt_FSM_Wrapper_Right/3(Steering_Chart_Substate) -> Data Store Write1/1
  Steering_Mgmt_FSM_Wrapper_Right/1(NMT_SendEnable) -> NMT_Enable_Right/1
  Steering_Mgmt_FSM_Wrapper_Right/2(SDO_SendEnable) -> SDO_Enable_Right/1
  Steering_Mgmt_FSM_Wrapper_Right/4(SDO_DataToSend) -> SDO_Data_Out_Right/1
  Steering_Mgmt_FSM_Wrapper_Right/5(PDO_SendEnable) -> AND/2, PDO_Enable_Right/1
  Steering_Mgmt_FSM_Wrapper_Right/6(Steering_Chart_State) -> Min/2
  Steering_Mgmt_FSM_Wrapper_Right/7(Steering_Best_Position) -> Steering_Best_Position_Right/1
  Min/1 -> SteeringState/1
  Steering_Mgmt_FSM_Wrapper_Left/8(Steering_Fault_Boolean) -> OR/1
  Amp Status Word Left/1 -> Steering_Mgmt_FSM_Wrapper_Left/5(Amp_Status_Word)
  Amp Status Word Right/1 -> Steering_Mgmt_FSM_Wrapper_Right/5(Amp_Status_Word)
  Steering_Mgmt_FSM_Wrapper_Left/5(PDO_SendEnable) -> NOT/1, SYNC Enable Left/1, PDO_Enable_Left/1
  AND/1 -> SYNC Enable Right/1
  NOT/1 -> AND/1
  Steering_Mgmt_FSM_Wrapper_Right/8(Steering_Fault_Boolean) -> OR/2
